simulink model "example2"  (Simulink 6.5)
settings: Solver=ode45  StartTime=0.0  StopTime=2  RelTol=1e-3
libraries: simulink_extras x1
settings Model: Creator=2414589  LastModifiedBy=2414589
settings DebuggingCC: MultiTaskDSMMsg=warning  MultiTaskCondExecSysMsg=none  StrictBusMsg=None
settings RTWCC: IncludeERTFirstTime=on

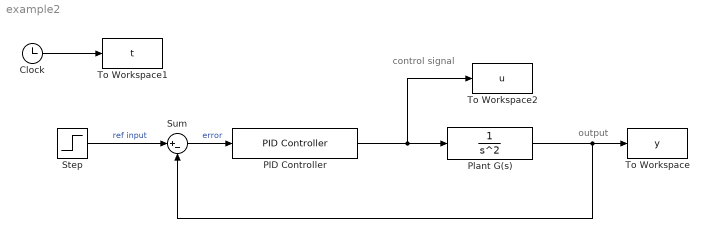
== system example2 ==
  note: control signal
  note: output
  Clock : Clock
      settings: Decimation=10
  PID Controller : simulink_extras/Additional Linear/PID Controller  SystemSampleTime=-1  P=1000  I=0  D=25
  Plant G(s) : TransferFcn  Numerator=1  Denominator=[1 0 0]
  Step : Step  Time=0  SampleTime=0
  Sum : Sum  Inputs=|+-
  To Workspace : ToWorkspace  VariableName=y  SampleTime=-1  SaveFormat=Array
  To Workspace1 : ToWorkspace  VariableName=t  SampleTime=-1  SaveFormat=Array
  To Workspace2 : ToWorkspace  VariableName=u  SampleTime=-1  SaveFormat=Array
  wires:
  Step/1 -> Sum/1  "ref input"
  Sum/1 -> PID Controller/1  "error"
  PID Controller/1 -> To Workspace2/1, Plant G(s)/1
  Plant G(s)/1 -> Sum/2, To Workspace/1
  Clock/1 -> To Workspace1/1
